simulink model "sim_pos_block"  (R2015a)
settings: Solver=ode3  StartTime=0.0  StopTime=7  FixedStep=0.01  RelTol=1e-3
undefined symbols (not defined in the file or in its folder): B, g, Grx, Ip, jp, l, mp, rrx
libraries: cstblocks x15, simulink x10
settings Model: Creator=Steffan  LastModifiedBy=Steffan

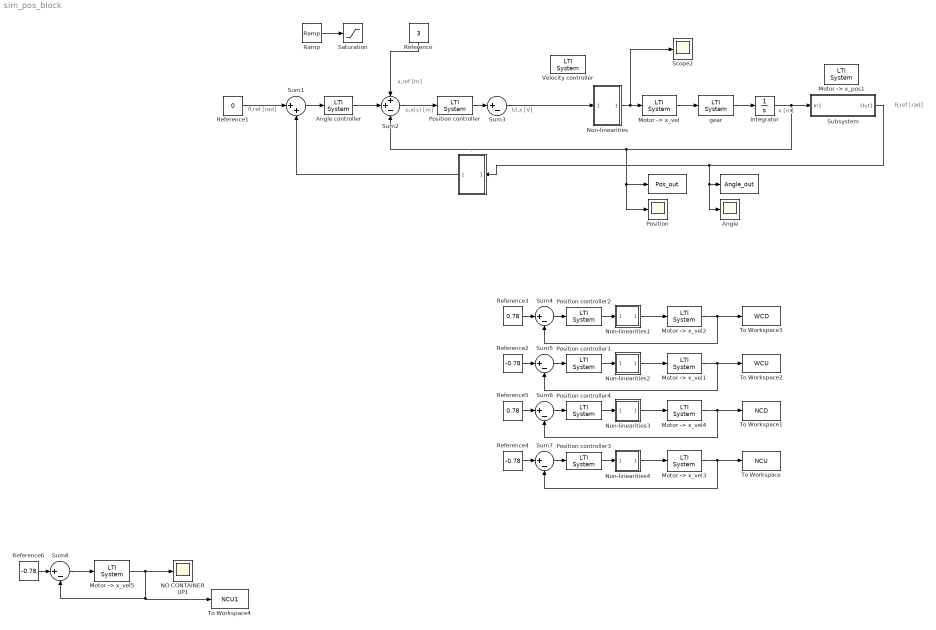
== system sim_pos_block ==
  note: θ,ref [rad]
  note: x [m]
  note: Ui,x [V]
  note: e,x(s) [m]
  note: x,ref [m]
  note: θ,ref [rad]
  " " : ToWorkspace  VariableName=Pos_out  SaveFormat=Timeseries  SampleTime=-1
  "  " : ToWorkspace  VariableName=Angle_out  SaveFormat=Timeseries  SampleTime=-1
  . : Subsystem
  Angle : Scope
      settings: YMin=-0.065  YMax=0.025
  Angle controller : cstblocks/LTI System  sys=Ppos  IC=[]
  Integrator : Integrator
  "Motor -> x_pos1" : cstblocks/LTI System  sys=W  IC=[]
  "Motor -> x_vel" : cstblocks/LTI System  sys=Mx  IC=[]
  "Motor -> x_vel1" : cstblocks/LTI System  sys=Hywu  IC=[]
  "Motor -> x_vel2" : cstblocks/LTI System  sys=Hywd  IC=[]
  "Motor -> x_vel3" : cstblocks/LTI System  sys=Hynu  IC=[]
  "Motor -> x_vel4" : cstblocks/LTI System  sys=Hynd  IC=[]
  "Motor -> x_vel5" : cstblocks/LTI System  sys=Mynu  IC=[]
  NO CONTAINER UP1 : Scope
      settings: YMin=-0.065  YMax=0.025  SaveName=ScopeData11
  Non-linearities : Subsystem
  Non-linearities1 : Subsystem
  Non-linearities2 : Subsystem
  Non-linearities3 : Subsystem
  Non-linearities4 : Subsystem
  Position : Scope
  Position controller : cstblocks/LTI System  sys=Ppos  IC=[]
  Position controller1 : cstblocks/LTI System  sys=Pywu  IC=[]
  Position controller2 : cstblocks/LTI System  sys=Pywd  IC=[]
  Position controller3 : cstblocks/LTI System  sys=Pynu  IC=[]
  Position controller4 : cstblocks/LTI System  sys=Pynd  IC=[]
  Ramp : simulink/Sources/Ramp  slope=0.5  start=0  X0=0
  Reference : Constant  Value=3
  Reference1 : Constant  Value=0
  Reference2 : Constant  Value=-0.78
  Reference3 : Constant  Value=0.78
  Reference4 : Constant  Value=-0.78
  Reference5 : Constant  Value=0.78
  Reference6 : Constant  Value=-0.78
  Saturation : Saturate  UpperLimit=3  LowerLimit=0
  Scope2 : Scope
      settings: YMin=-0.065  YMax=0.025  SaveName=ScopeData2
  Subsystem : Subsystem
  Sum1 : Sum  Inputs=|++
  Sum2 : Sum  Inputs=++-
  Sum{3..8} (6 alike) : Sum  Inputs=|+-
  To Workspace : ToWorkspace  VariableName=NCU  SaveFormat=Timeseries  SampleTime=-1
  To Workspace1 : ToWorkspace  VariableName=NCD  SaveFormat=Timeseries  SampleTime=-1
  To Workspace2 : ToWorkspace  VariableName=WCU  SaveFormat=Timeseries  SampleTime=-1
  To Workspace3 : ToWorkspace  VariableName=WCD  SaveFormat=Timeseries  SampleTime=-1
  To Workspace4 : ToWorkspace  VariableName=NCU1  SaveFormat=Timeseries  SampleTime=-1
  Velocity controller : cstblocks/LTI System  sys=Pvel  IC=[]
  gear : cstblocks/LTI System  sys=Grx*rrx  IC=[]
  wires:
  "Motor -> x_vel"/1 -> gear/1
  Sum2/1 -> Position controller/1
  Reference/1 -> Sum2/1
  Reference1/1 -> Sum1/1
  Sum1/1 -> Angle controller/1
  Angle controller/1 -> Sum2/2
  ./1(Out1) -> Sum1/2
  Position controller/1 -> Sum3/1
  Non-linearities/1(Out1) -> Scope2/1, "Motor -> x_vel"/1
  gear/1 -> Integrator/1
  Subsystem/1(Out1) -> ./1(In1), Angle/1, "  "/1
  Integrator/1 -> Subsystem/1(In1), Sum2/3, Position/1, " "/1
  Ramp/1 -> Saturation/1
  Sum3/1 -> Non-linearities/1(In1)
  Sum4/1 -> Position controller2/1
  Reference3/1 -> Sum4/1
  "Motor -> x_vel2"/1 -> Sum4/2, To Workspace3/1
  Sum5/1 -> Position controller1/1
  Reference2/1 -> Sum5/1
  "Motor -> x_vel1"/1 -> Sum5/2, To Workspace2/1
  Position controller2/1 -> Non-linearities1/1(In1)
  Position controller1/1 -> Non-linearities2/1(In1)
  Sum6/1 -> Position controller4/1
  Reference5/1 -> Sum6/1
  "Motor -> x_vel4"/1 -> Sum6/2, To Workspace1/1
  Sum7/1 -> Position controller3/1
  Reference4/1 -> Sum7/1
  "Motor -> x_vel3"/1 -> Sum7/2, To Workspace/1
  Position controller4/1 -> Non-linearities3/1(In1)
  Position controller3/1 -> Non-linearities4/1(In1)
  Reference6/1 -> Sum8/1
  "Motor -> x_vel5"/1 -> NO CONTAINER UP1/1, To Workspace4/1, Sum8/2
  Sum8/1 -> "Motor -> x_vel5"/1
  Non-linearities1/1(Out1) -> "Motor -> x_vel2"/1
  Non-linearities2/1(Out1) -> "Motor -> x_vel1"/1
  Non-linearities3/1(Out1) -> "Motor -> x_vel4"/1
  Non-linearities4/1(Out1) -> "Motor -> x_vel3"/1

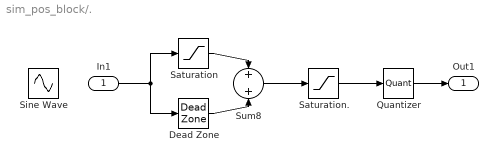
== system sim_pos_block/. ==
  In1 : Inport
  Dead Zone : DeadZone  LowerValue=-0.3387  UpperValue=0.3227  SaturateOnIntegerOverflow=on
  Quantizer : Quantizer  QuantizationInterval=0.001
  Saturation : Saturate  UpperLimit=.1627  LowerLimit=-0.1787
  Saturation. : Saturate  UpperLimit=0.664  LowerLimit=-0.68
  Sine Wave : Sin  SampleTime=0
  Sum8 : Sum  Inputs=+|+
  Out1 : Outport
  wires:
  Dead Zone/1 -> Sum8/2
  Saturation/1 -> Sum8/1
  Sum8/1 -> Saturation./1
  In1/1 -> Saturation/1, Dead Zone/1
  Saturation./1 -> Quantizer/1
  Quantizer/1 -> Out1/1

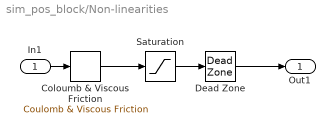
== system sim_pos_block/Non-linearities ==
  In1 : Inport
  Coloumb & Viscous Friction : simulink/Discontinuities/Coulomb & Viscous Friction  offset=[4.2]  gain=1
  Dead Zone : DeadZone  LowerValue=-4.2  UpperValue=4.2  SaturateOnIntegerOverflow=on
  Saturation : Saturate  UpperLimit=12.5  LowerLimit=-12.5
  Out1 : Outport
  wires:
  Dead Zone/1 -> Out1/1
  Saturation/1 -> Dead Zone/1
  Coloumb & Viscous Friction/1 -> Saturation/1
  In1/1 -> Coloumb & Viscous Friction/1

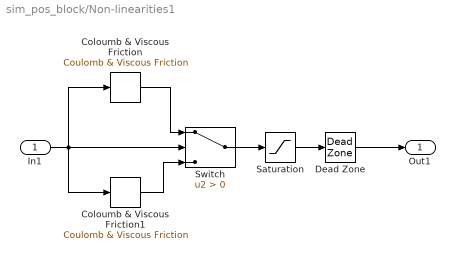
== system sim_pos_block/Non-linearities1 ==
  In1 : Inport
  Coloumb & Viscous Friction : simulink/Discontinuities/Coulomb & Viscous Friction  offset=[3]  gain=1
  Coloumb & Viscous Friction1 : simulink/Discontinuities/Coulomb & Viscous Friction  offset=[5.5]  gain=1
  Dead Zone : DeadZone  LowerValue=-5.5  UpperValue=3  SaturateOnIntegerOverflow=on
  Saturation : Saturate  UpperLimit=12.5  LowerLimit=-12.5
  Switch : Switch  Criteria=u2 > Threshold
  Out1 : Outport
  wires:
  Dead Zone/1 -> Out1/1
  Saturation/1 -> Dead Zone/1
  Switch/1 -> Saturation/1
  In1/1 -> Switch/2, Coloumb & Viscous Friction/1, Coloumb & Viscous Friction1/1
  Coloumb & Viscous Friction1/1 -> Switch/3
  Coloumb & Viscous Friction/1 -> Switch/1

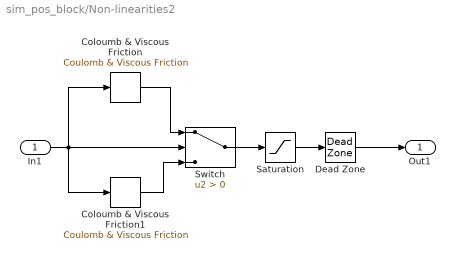
== system sim_pos_block/Non-linearities2 ==
  In1 : Inport
  Coloumb & Viscous Friction : simulink/Discontinuities/Coulomb & Viscous Friction  offset=[3]  gain=1
  Coloumb & Viscous Friction1 : simulink/Discontinuities/Coulomb & Viscous Friction  offset=[5.5]  gain=1
  Dead Zone : DeadZone  LowerValue=-5.5  UpperValue=3  SaturateOnIntegerOverflow=on
  Saturation : Saturate  UpperLimit=12.5  LowerLimit=-12.5
  Switch : Switch  Criteria=u2 > Threshold
  Out1 : Outport
  wires:
  Dead Zone/1 -> Out1/1
  Saturation/1 -> Dead Zone/1
  Switch/1 -> Saturation/1
  In1/1 -> Switch/2, Coloumb & Viscous Friction/1, Coloumb & Viscous Friction1/1
  Coloumb & Viscous Friction1/1 -> Switch/3
  Coloumb & Viscous Friction/1 -> Switch/1

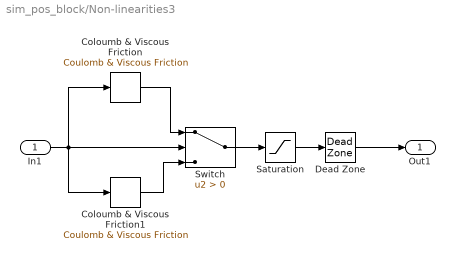
== system sim_pos_block/Non-linearities3 ==
  In1 : Inport
  Coloumb & Viscous Friction : simulink/Discontinuities/Coulomb & Viscous Friction  offset=[3]  gain=1
  Coloumb & Viscous Friction1 : simulink/Discontinuities/Coulomb & Viscous Friction  offset=[5.5]  gain=1
  Dead Zone : DeadZone  LowerValue=-5.5  UpperValue=3  SaturateOnIntegerOverflow=on
  Saturation : Saturate  UpperLimit=12.5  LowerLimit=-12.5
  Switch : Switch  Criteria=u2 > Threshold
  Out1 : Outport
  wires:
  Dead Zone/1 -> Out1/1
  Saturation/1 -> Dead Zone/1
  Switch/1 -> Saturation/1
  In1/1 -> Switch/2, Coloumb & Viscous Friction/1, Coloumb & Viscous Friction1/1
  Coloumb & Viscous Friction1/1 -> Switch/3
  Coloumb & Viscous Friction/1 -> Switch/1

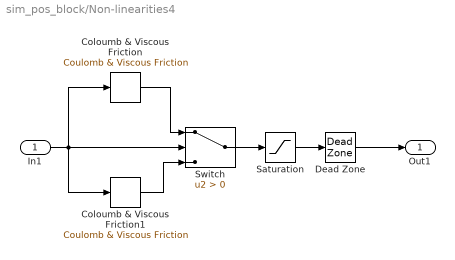
== system sim_pos_block/Non-linearities4 ==
  In1 : Inport
  Coloumb & Viscous Friction : simulink/Discontinuities/Coulomb & Viscous Friction  offset=[3]  gain=1
  Coloumb & Viscous Friction1 : simulink/Discontinuities/Coulomb & Viscous Friction  offset=[5.5]  gain=1
  Dead Zone : DeadZone  LowerValue=-5.5  UpperValue=3  SaturateOnIntegerOverflow=on
  Saturation : Saturate  UpperLimit=12.5  LowerLimit=-12.5
  Switch : Switch  Criteria=u2 > Threshold
  Out1 : Outport
  wires:
  Dead Zone/1 -> Out1/1
  Saturation/1 -> Dead Zone/1
  Switch/1 -> Saturation/1
  In1/1 -> Switch/2, Coloumb & Viscous Friction/1, Coloumb & Viscous Friction1/1
  Coloumb & Viscous Friction1/1 -> Switch/3
  Coloumb & Viscous Friction/1 -> Switch/1

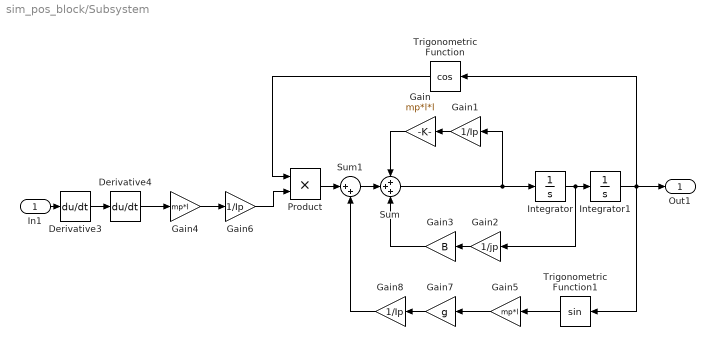
== system sim_pos_block/Subsystem ==
  In1 : Inport
  Derivative3 : Derivative
  Derivative4 : Derivative
  Gain : Gain  Gain=mp*l*l
  Gain1 : Gain  Gain=1/Ip
  Gain2 : Gain  Gain=1/jp
  Gain3 : Gain  Gain=B
  Gain4 : Gain  Gain=mp*l
  Gain5 : Gain  Gain=mp*l
  Gain6 : Gain  Gain=1/Ip
  Gain7 : Gain  Gain=g
  Gain8 : Gain  Gain=1/Ip
  Integrator : Integrator
  Integrator1 : Integrator
  Product : Product
  Sum : Sum  Inputs=+++
  Sum1 : Sum  Inputs=|++
  Trigonometric Function : Trigonometry  Operator=cos
  Trigonometric Function1 : Trigonometry
  Out1 : Outport
  wires:
  Sum/1 -> Gain1/1, Integrator/1
  Integrator/1 -> Gain2/1, Integrator1/1
  Gain/1 -> Sum/1
  Gain1/1 -> Gain/1
  Gain2/1 -> Gain3/1
  Gain3/1 -> Sum/3
  Integrator1/1 -> Out1/1, Trigonometric Function1/1, Trigonometric Function/1
  Derivative3/1 -> Derivative4/1
  Derivative4/1 -> Gain4/1
  Product/1 -> Sum1/1
  Trigonometric Function/1 -> Product/1
  Gain4/1 -> Gain6/1
  Gain6/1 -> Product/2
  Trigonometric Function1/1 -> Gain5/1
  Gain5/1 -> Gain7/1
  Gain7/1 -> Gain8/1
  Gain8/1 -> Sum1/2
  Sum1/1 -> Sum/2
  In1/1 -> Derivative3/1
